simulink library "airlib"  (Simulink 3.00)
libraries: airlib x2
(part 1 of 2)
settings Model: LastModifiedBy=campa

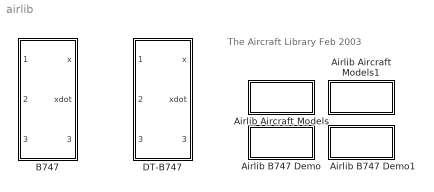
== system airlib ==
  note: The Aircraft Library
      | Feb 2003
  Airlib Aircraft Models : Subsystem
      settings: OpenFcn=airlibex
      mask Display: disp('Aircraft\nModels')
  Airlib Aircraft Models1 : Subsystem
      settings: OpenFcn=airgk
      mask Display: disp('General\nController')
  Airlib B747 Demo : Subsystem
      settings: OpenFcn=B747cl
      mask Display: disp('B747\nClosed Loop')
  Airlib B747 Demo1 : Subsystem
      settings: OpenFcn=fdcwind
      mask Display: disp('FDC\nwind model')
  B747 : Subsystem  mask(General Nonlinear Aircraft Model){GM1=[8.32   59.74   510.95   24675560  44876980   67383260   0   1315126  0   288772], CD_wind=[0.0164  0.2  0  0  0], CL_wind=[0.21  4.4  6.6  0.32  0.7], Cm_body=[0  -1   -20.5    -1.3    -2.7], CY_body=[0   -0.9    0     0     -0    0.12], Cl_body=[0    -0.16    -0.34   0.13    -0.013    0.008], Cn_body=[0    0.16   -0.026    -0.28     -0.0018   -0.1], x0=[150.148  0.0464959 0   0 0 0   0 0.0464959 0   0 0 61]}
      mask prompts: GM1 "Geometry and Mass : [cbar   b    S    Ix   Iy   Iz   Jxy  Jxz  Jyz  m]"; CD_wind "Aerodynamic D-Force Derivatives : [CD0 CDa CDq CDde CDih]"; CL_wind "Aerodynamic L-Force Derivatives : [CL0 CLa CLq CLde CLih]"; Cm_body "Aerodynamic Y-Moment Derivatives : [Cm0 Cma Cmq Cmde Cmih]"; CY_body "Aerodynamic Y-Force Derivatives : [CY0 CYb CYp CYr CYda CYdr]"; Cl_body "Aerodynamic X-moment Derivatives : [Cl0 Clb Clp Clr Clda Cldr]"; Cn_body "Aerodynamic Z-moment Derivatives : [Cn0 Cnb Cnp Cnr Cnda Cndr]"; x0 "Initial Condition x0 [v alpha beta p q r psi theta phi xe ye H]"
      mask help:
      | The first input contains the wind velocity and acceleration.
      |   The second input contains external forces and moments in body axis.
      |   The third input contains the deflections of elevators, ailerons, rudder,
      |   and flaps. For a list of outputs look under the mask.
      |   NB : The International measurement system (MKS) is adopted.
      mask init:
      | AM=zeros(6,19);
      | AM(1,[1 2 9 11 12])=reshape(CD_wind,1,5);
      | AM(3,[1 2 9 11 12])=reshape(CL_wind,1,5);
      | AM(5,[1 2 9 11 12])=reshape(Cm_body,1,5);
      | AM(2,[1 5 8 10 13 14])=reshape(CY_body,1,6);
      | AM(4,[1 5 8 10 13 14])=reshape(Cl_body,1,6);
      | AM(6,[1 5 8 10 13 14])=reshape(Cn_body,1,6);
      | 
      | Ix=GM1(4);Iy=GM1(5);Iz=GM1(6);
      | Jxy=GM1(7);Jxz=GM1(8);Jyz=GM1(9);
      | 
      | detI = Ix*Iy*Iz - 2*Jxy*Jxz*Jyz - Ix*Jyz^2 - Iy*Jxz^2 - Iz*Jxy^2;
      | I1   = Iy*Iz - Jyz^2;I2   = Jxy*Iz + Jyz*Jxz;
      | I3   = Jxy*Jyz + Iy*Jxz;I4   = Ix*Iz - Jxz^2;
      | I5   = Ix*Jyz + Jxy*Jxz;I6   = Ix*Iy - Jxy^2;
      | 
      | Pl  = I1/detI; Pm = I2/detI; Pn = I3/detI;
      | Ppp = -(Jxz*I2 - Jxy*I3)/detI;Ppq = (Jxz*I1 - Jyz*I2 - (Iy-Ix)*I3)/detI;
      | Ppr = -(Jxy*I1 + (Ix-Iz)*I2 - Jyz*I3)/detI;Pqq = (Jyz*I1 - Jxy*I3)/detI;
      | Pqr = -((Iz-Iy)*I1 - Jxy*I2 + Jxz*I3)/detI;Prr = -(Jyz*I1 - Jxz*I2)/detI;
      | 
      | Ql  = I2/detI; Qm = I4/detI; Qn = I5/detI;
      | Qpp = -(Jxz*I4 - Jxy*I5)/detI;Qpq = (Jxz*I2 - Jyz*I4 - (Iy-Ix)*I5)/detI;
      | Qpr = -(Jxy*I2 + (Ix-Iz)*I4 - Jyz*I5)/detI;Qqq = (Jyz*I2 - Jxy*I5)/detI;
      | Qqr = -((Iz-Iy)*I2 - Jxy*I4 + Jxz*I5)/detI;Qrr = -(Jyz*I2 - Jxz*I4)/detI;
      | 
      | Rl  = I3/detI; Rm = I5/detI; Rn = I6/detI;
      | Rpp = -(Jxz*I5 - Jxy*I6)/detI;
      | Rpq = (Jxz*I3 - Jyz*I5 - (Iy-Ix)*I6)/detI;
      | Rpr = -(Jxy*I3 + (Ix-Iz)*I5 - Jyz*I6)/detI;
      | Rqq = (Jyz*I3 - Jxy*I6)/detI;
      | Rqr = -((Iz-Iy)*I3 - Jxy*I5 + Jxz*I6)/detI;
      | Rrr = -(Jyz*I3 - Jxz*I5)/detI;
      | 
      | GM2 = [  Pl   Pm   Pn   Ppp  Ppq  Ppr  Pqq  Pqr  Prr ;
      |                Ql  Qm   Qn   Qpp  Qpq  Qpr  Qqq  Qqr  Qrr ;
      |                Rl  Rm   Rn   Rpp  Rpq  Rpr  Rqq  Rqr  Rrr ];
      | 
      | xfix=1;
      mask Help:
      | <p>
      | This block is a general nonlinear 6DOF aircraft model, with a very accurate built-in atmosphere model and constant aerodynamic derivatives.
      | The architecture of the block is largely based on the Aircraft block provided by the <A
      | HREF="http://www.mathworks.com/matlabcentral/fileexchange/loadFile.do?objectId=252&objectType=file">FDC toolbox</A> (Marc Rauw, 1993-2000).
      | </p>
      | <p>
      | The geometric and inertal data of the aircraft are entered as parameters in the first row of the mask. The other six rows contains the
      | non-dimensional aerodynamic derivatives. The last row is the initial state.
      | </p>
      | <p>
      | The first input contains the wind velocity and acceleration.
      | The second input contains external forces and moments in the aircraft body axis.
      | The third input contains the deflections of elevators, ailerons, rudder,
      | and flaps or stabilators. For a list of outputs look under the mask.
      | </p>
      | <p>
      | The control surface sign conventions are the same adopted in books such as Stevens-Lewis and Etkin, and in many flight simulators,
      | including the FDC toolbox. <br>
      | Specifically, positive elevator deflection causes negative pitching moment (Cmde &#60 0), positive rudder deflection causes negative yawing
      | moment (Cndr &#60 0), and positive aileron deflection causes negative rolling moment (Clda &#60 0). Another way to say the same thing is
      | that, the positive elevators deflection is Trailing Edge Down (TED), the positive rudder(s) deflection is Trailing Edge Left (TEL), and,
      | taking as TED the positive ailerons deflection, da=K*(da_right-da_left), with K usually equal to 1 (FDC) or 1/2.
      | </p>
      | <p>
      | Since this block is largely based on the FDC toolbox, i redirect you to the FDC Toolbox manual, for a good explanation of the underlying
      | components. Besides the mask and the fact that the aerodynamic derivatives are expressed in the stability axis, the only relevant difference
      | with the FDC toolbox is that in the computation of the aerodynamic forces, q is normalized as q*cbar/2V instead of q*cbar/V. The majority
      | of aeronautics books that i've seen use q*cbar/2V.
      | </p>
      | <p>
      | Please note that the International Measurement System is adopted. So, lengths are in meters, masses in Kg, and inertia moments in Kg*m^2.
      | Moreover, forces are in N, moments in N*m, accelerations in g, and angles in radians. For those that use the english system, here are some useful
      | conversion factors: <br>
      | 1 ft   = 0.3048 m, 1 lb   = 0.4536 Kg, 1 slug = 14.593903 Kg ,  1 slug*ft^2 = 1.355818 Kg*m^2
      | <br>
      | </p>
      | <p>
      | Finally, there is an <A HREF="http://www.aae.uiuc.edu/m-selig/apasim/Aircraft-uiuc.html">excellent source</A> of aircraft aerodynamic data
      | which is mantained by Michael S. Selig, Rob Deters, and Glen Dimock at the university of Urbana-Champaign. To use any of the given models
      | you just need to type the supplied aircraft data in the block mask.
      | </p>
      | <p>
      | <p>
      | December 2002, Giampiero Campa
      | </p>
      | </p>
      mask Display: disp('General\nAircraft\nModel')
  DT-B747 : Subsystem  mask(Discrete Time General Nonlinear Aircraft Model){GM1=[8.32   59.74   510.95   24675560  44876980   67383260   0   1315126  0   288772  0.05], CD_wind=[0.0164  0.2  0  0  0], CL_wind=[0.21  4.4  6.6  0.32  0.7], Cm_body=[0  -1   -20.5    -1.3    -2.7], CY_body=[0   -0.9    0     0     -0    0.12], Cl_body=[0    -0.16    -0.34   0.13    -0.013    0.008], Cn_body=[0    0.16   -0.026    -0.28     -0.0018   -0.1], x0=[150.148  0.0464959 0   0 0 0   0 0.0464959 0   0 0 61]}
      mask prompts: GM1 "Geometry, Mass, T : [cbar   b    S    Ix   Iy   Iz   Jxy  Jxz  Jyz  m  T]"; CD_wind "Aerodynamic D-Force Derivatives : [CD0 CDa CDq CDde CDih]"; CL_wind "Aerodynamic L-Force Derivatives : [CL0 CLa CLq CLde CLih]"; Cm_body "Aerodynamic Y-Moment Derivatives : [Cm0 Cma Cmq Cmde Cmih]"; CY_body "Aerodynamic Y-Force Derivatives : [CY0 CYb CYp CYr CYda CYdr]"; Cl_body "Aerodynamic X-moment Derivatives : [Cl0 Clb Clp Clr Clda Cldr]"; Cn_body "Aerodynamic Z-moment Derivatives : [Cn0 Cnb Cnp Cnr Cnda Cndr]"; x0 "Initial Condition x0 [v alpha beta p q r psi theta phi xe ye H]"
      mask help:
      | The first input contains the wind velocity and acceleration.
      |   The second input contains external forces and moments in body axis.
      |   The third input contains the deflections of elevators, ailerons, rudder,
      |   and flaps. For a list of outputs look under the mask.
      |   NB : The International measurement system (MKS) is adopted.
      mask init:
      | AM=zeros(6,19);
      | AM(1,[1 2 9 11 12])=reshape(CD_wind,1,5);
      | AM(3,[1 2 9 11 12])=reshape(CL_wind,1,5);
      | AM(5,[1 2 9 11 12])=reshape(Cm_body,1,5);
      | AM(2,[1 5 8 10 13 14])=reshape(CY_body,1,6);
      | AM(4,[1 5 8 10 13 14])=reshape(Cl_body,1,6);
      | AM(6,[1 5 8 10 13 14])=reshape(Cn_body,1,6);
      | 
      | Ix=GM1(4);Iy=GM1(5);Iz=GM1(6);
      | Jxy=GM1(7);Jxz=GM1(8);Jyz=GM1(9);
      | 
      | detI = Ix*Iy*Iz - 2*Jxy*Jxz*Jyz - Ix*Jyz^2 - Iy*Jxz^2 - Iz*Jxy^2;
      | I1   = Iy*Iz - Jyz^2;I2   = Jxy*Iz + Jyz*Jxz;
      | I3   = Jxy*Jyz + Iy*Jxz;I4   = Ix*Iz - Jxz^2;
      | I5   = Ix*Jyz + Jxy*Jxz;I6   = Ix*Iy - Jxy^2;
      | 
      | Pl  = I1/detI; Pm = I2/detI; Pn = I3/detI;
      | Ppp = -(Jxz*I2 - Jxy*I3)/detI;Ppq = (Jxz*I1 - Jyz*I2 - (Iy-Ix)*I3)/detI;
      | Ppr = -(Jxy*I1 + (Ix-Iz)*I2 - Jyz*I3)/detI;Pqq = (Jyz*I1 - Jxy*I3)/detI;
      | Pqr = -((Iz-Iy)*I1 - Jxy*I2 + Jxz*I3)/detI;Prr = -(Jyz*I1 - Jxz*I2)/detI;
      | 
      | Ql  = I2/detI; Qm = I4/detI; Qn = I5/detI;
      | Qpp = -(Jxz*I4 - Jxy*I5)/detI;Qpq = (Jxz*I2 - Jyz*I4 - (Iy-Ix)*I5)/detI;
      | Qpr = -(Jxy*I2 + (Ix-Iz)*I4 - Jyz*I5)/detI;Qqq = (Jyz*I2 - Jxy*I5)/detI;
      | Qqr = -((Iz-Iy)*I2 - Jxy*I4 + Jxz*I5)/detI;Qrr = -(Jyz*I2 - Jxz*I4)/detI;
      | 
      | Rl  = I3/detI; Rm = I5/detI; Rn = I6/detI;
      | Rpp = -(Jxz*I5 - Jxy*I6)/detI;
      | Rpq = (Jxz*I3 - Jyz*I5 - (Iy-Ix)*I6)/detI;
      | Rpr = -(Jxy*I3 + (Ix-Iz)*I5 - Jyz*I6)/detI;
      | Rqq = (Jyz*I3 - Jxy*I6)/detI;
      | Rqr = -((Iz-Iy)*I3 - Jxy*I5 + Jxz*I6)/detI;
      | Rrr = -(Jyz*I3 - Jxz*I5)/detI;
      | 
      | GM2 = [  Pl   Pm   Pn   Ppp  Ppq  Ppr  Pqq  Pqr  Prr ;
      |                Ql  Qm   Qn   Qpp  Qpq  Qpr  Qqq  Qqr  Qrr ;
      |                Rl  Rm   Rn   Rpp  Rpq  Rpr  Rqq  Rqr  Rrr ];
      | 
      | xfix=1;
      | T=GM1(11);
      mask Help:
      | <p>
      | This block is a general nonlinear 6DOF aircraft model, with a very accurate built-in atmosphere model and constant aerodynamic derivatives.
      | The architecture of the block is largely based on the Aircraft block provided by the <A
      | HREF="http://www.mathworks.com/matlabcentral/fileexchange/loadFile.do?objectId=252&objectType=file">FDC toolbox</A> (Marc Rauw, 1993-2000).
      | </p>
      | <p>
      | The geometric and inertal data of the aircraft are entered as parameters in the first row of the mask, sampling time is the last parameter. The other six rows contains the non-dimensional aerodynamic derivatives. The last row is the initial state.
      | </p>
      | <p>
      | The first input contains the wind velocity and acceleration.
      | The second input contains external forces and moments in the aircraft body axis.
      | The third input contains the deflections of elevators, ailerons, rudder,
      | and flaps or stabilators. For a list of outputs look under the mask.
      | </p>
      | <p>
      | The control surface sign conventions are the same adopted in books such as Stevens-Lewis and Etkin, and in many flight simulators,
      | including the FDC toolbox. <br>
      | Specifically, positive elevator deflection causes negative pitching moment (Cmde &#60 0), positive rudder deflection causes negative yawing
      | moment (Cndr &#60 0), and positive aileron deflection causes negative rolling moment (Clda &#60 0). Another way to say the same thing is
      | that, the positive elevators deflection is Trailing Edge Down (TED), the positive rudder(s) deflection is Trailing Edge Left (TEL), and,
      | taking as TED the positive ailerons deflection, da=K*(da_right-da_left), with K usually equal to 1 (FDC) or 1/2.
      | </p>
      | <p>
      | Since this block is largely based on the FDC toolbox, i redirect you to the FDC Toolbox manual, for a good explanation of the underlying
      | components. Besides the mask and the fact that the aerodynamic derivatives are expressed in the stability axis, the only relevant difference
      | with the FDC toolbox is that in the computation of the aerodynamic forces, q is normalized as q*cbar/2V instead of q*cbar/V. The majority
      | of aeronautics books that i've seen use q*cbar/2V.
      | </p>
      | <p>
      | Please note that the International Measurement System is adopted. So, lengths are in meters, masses in Kg, and inertia moments in Kg*m^2.
      | Moreover, forces are in N, moments in N*m, accelerations in g, and angles in radians. For those that use the english system, here are some useful
      | conversion factors: <br>
      | 1 ft   = 0.3048 m, 1 lb   = 0.4536 Kg, 1 slug = 14.593903 Kg ,  1 slug*ft^2 = 1.355818 Kg*m^2
      | <br>
      | </p>
      | <p>
      | Finally, there is an <A HREF="http://www.aae.uiuc.edu/m-selig/apasim/Aircraft-uiuc.html">excellent source</A> of aircraft aerodynamic data
      | which is mantained by Michael S. Selig, Rob Deters, and Glen Dimock at the university of Urbana-Champaign. To use any of the given models
      | you just need to type the supplied aircraft data in the block mask.
      | </p>
      | <p>
      | <p>
      | December 2002, Giampiero Campa
      | </p>
      | </p>
      mask Display: disp('Discrete\nTime\nGeneral\nAircraft\nModel')

== system airlib/Airlib Aircraft Models ==

== system airlib/Airlib Aircraft Models1 ==

== system airlib/Airlib B747 Demo ==

== system airlib/Airlib B747 Demo1 ==

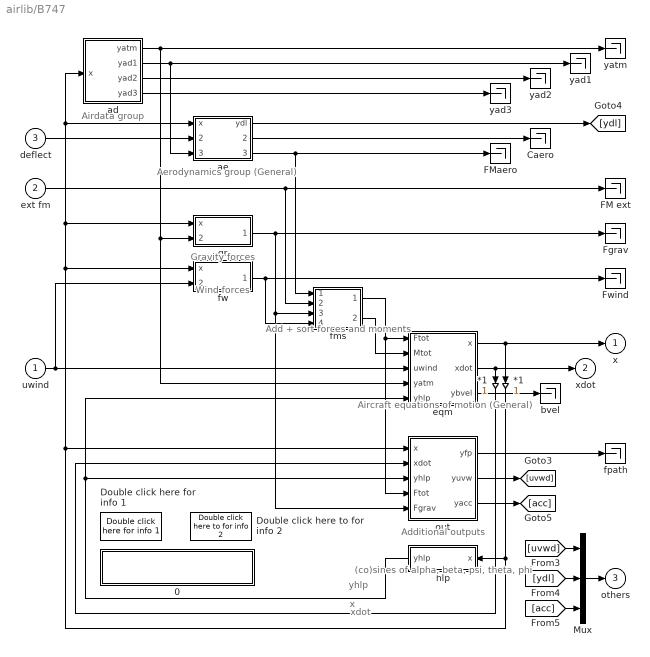
== system airlib/B747 ==
  note: Airdata group
  note: Add + sort
      | forces and
      | moments
  note: (co)sines of
      | alpha, beta,
      | psi, theta, phi
  note: Aerodynamics
      | group (General)
  note: Gravity forces
  note: Wind forces
  note: Aircraft equations
      | of motion (General)
  note: Additional outputs
  note: yhlp
  note: x
  note: xdot
  " uwind" : Inport  Port=1  PortWidth=-1  SampleTime=-1  DataType=auto
      settings: SignalType=auto
  ext fm : Inport  Port=2  PortWidth=-1  SampleTime=-1  DataType=auto
      settings: SignalType=auto
  deflect : Inport  Port=3  PortWidth=-1  SampleTime=-1  DataType=auto
      settings: SignalType=auto
  " *1" : Gain  Orientation=down  Gain=1  SaturateOnIntegerOverflow=on
  *1 : Gain  Orientation=down  Gain=1  SaturateOnIntegerOverflow=on
  0 : Subsystem
      mask Display: disp('AIRCRAFT, main level\nM.O. Rauw')
  Caero : Terminator
  Double click here for info 1 : airlib/DT-B747/Double click here for info 1
  Double click here to for info 2 : airlib/DT-B747/Double click here to for info 2
  FM ext : Terminator
  FMaero : Terminator
  Fgrav : Terminator
  Fwind : Terminator
  Mux : Mux  Inputs=[3 3 6]
  ad : Subsystem
  ae : Subsystem
  bvel : Terminator
  eqm : Subsystem
  fms : Subsystem
      mask Type: FMsort
      mask Description: Forces and Moments sorting block
      mask Display: disp('FMsort')
  fpath : Terminator
  fw : Subsystem  mask(fwind){m=GM1(10)}
      mask prompts: m "Mass of the aircraft [kg]:"
      mask help: Forces due to non-steady atmosphere.
      mask Display: disp('Fwind')
  gr : Subsystem  mask(Gravity){m=GM1(10)}
      mask prompts: m "Mass of the aircraft [kg]:"
      mask help: Gravity forces.
      mask Display: disp('Gravity')
  hlp : Subsystem  Orientation=left
      mask Type: Hlpfcn
      mask Description: Help sines and cosines
      mask Display: disp('hlpfcn')
  out : Subsystem
  yad1 : Terminator
  yad2 : Terminator
  yad3 : Terminator
  yatm : Terminator
  x : Outport  Port=1
  xdot : Outport  Port=2
  others : Outport  Port=3
  wires:
  Mux/1 -> others/1
  [acc] -> Mux/3
  [ydl] -> Mux/2
  [uvwd] -> Mux/1
  out/2(yuvw) -> [uvwd]
  fms/2(Mtot) -> eqm/2(Mtot)
  eqm/1(x) -> " *1"/1, x/1
  eqm/2(xdot) -> *1/1, xdot/1
  " *1"/1 -> ad/1(x), ae/1(x), gr/1(x), fw/1(x), out/1(x), hlp/1(x)
  gr/1(Fgrav) -> Fgrav/1, out/5(Fgrav), fms/3(Fgrav)
  *1/1 -> out/2(xdot)
  " uwind"/1 -> fw/2(uwind), eqm/3(uwind)
  hlp/1(yhlp) -> out/3(yhlp), eqm/5(yhlp)
  ae/3(FMaero) -> fms/1(FMaero), FMaero/1
  fw/1(Fwind) -> fms/4(Fwind), Fwind/1
  out/3(yacc) -> [acc]
  ad/1(yatm) -> yatm/1, gr/2(yatm), eqm/4(yatm)
  ad/3(yad2) -> yad2/1
  ad/2(yad1) -> yad1/1, ae/3(yad1)
  out/1(yfp) -> fpath/1
  eqm/3(ybvel) -> bvel/1
  ae/2(Caero) -> Caero/1
  ae/1(ydl) -> [ydl]
  ad/4(yad3) -> yad3/1
  deflect/1 -> ae/2(uaero)
  ext fm/1 -> FM ext/1, fms/2(FMprop)
  fms/1(Ftot) -> eqm/1(Ftot), out/4(Ftot)

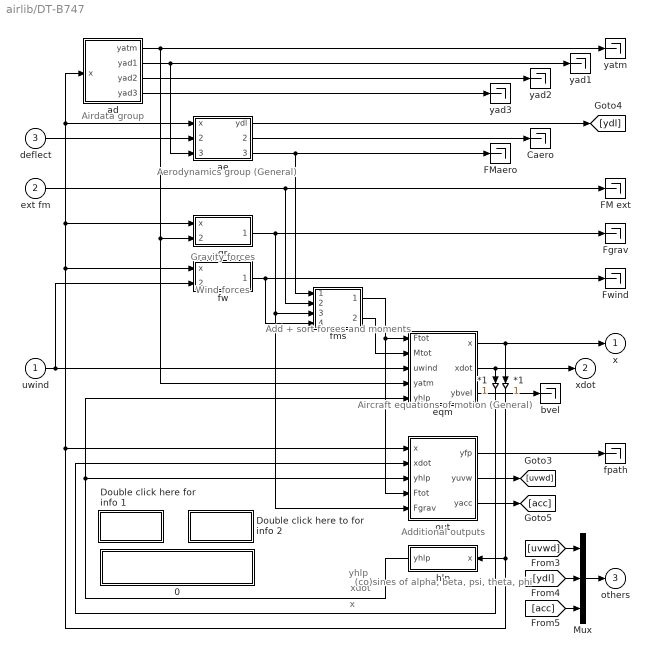
== system airlib/DT-B747 ==
  note: xdot
  note: x
  note: yhlp
  note: Additional outputs
  note: Aircraft equations
      | of motion (General)
  note: Wind forces
  note: Gravity forces
  note: Aerodynamics
      | group (General)
  note: (co)sines of
      | alpha, beta,
      | psi, theta, phi
  note: Add + sort
      | forces and
      | moments
  note: Airdata group
  " uwind" : Inport  Port=1  PortWidth=-1  SampleTime=-1  DataType=auto
      settings: SignalType=auto
  ext fm : Inport  Port=2  PortWidth=-1  SampleTime=-1  DataType=auto
      settings: SignalType=auto
  deflect : Inport  Port=3  PortWidth=-1  SampleTime=-1  DataType=auto
      settings: SignalType=auto
  " *1" : Gain  Orientation=down  Gain=1  SaturateOnIntegerOverflow=on
  *1 : Gain  Orientation=down  Gain=1  SaturateOnIntegerOverflow=on
  0 : Subsystem
      mask Display: disp('AIRCRAFT, main level\nM.O. Rauw')
  Caero : Terminator
  Double click here for info 1 : Subsystem
      mask Display: disp('Input\nSignals')
  Double click here to for info 2 : Subsystem
      mask Display: disp('Output\nSignals')
  FM ext : Terminator
  FMaero : Terminator
  Fgrav : Terminator
  Fwind : Terminator
  Mux : Mux  Inputs=[3 3 6]
  ad : Subsystem
  ae : Subsystem
  bvel : Terminator
  eqm : Subsystem
  fms : Subsystem
      mask Type: FMsort
      mask Description: Forces and Moments sorting block
      mask Display: disp('FMsort')
  fpath : Terminator
  fw : Subsystem  mask(fwind){m=GM1(10)}
      mask prompts: m "Mass of the aircraft [kg]:"
      mask help: Forces due to non-steady atmosphere.
      mask Display: disp('Fwind')
  gr : Subsystem  mask(Gravity){m=GM1(10)}
      mask prompts: m "Mass of the aircraft [kg]:"
      mask help: Gravity forces.
      mask Display: disp('Gravity')
  hlp : Subsystem  Orientation=left
      mask Type: Hlpfcn
      mask Description: Help sines and cosines
      mask Display: disp('hlpfcn')
  out : Subsystem
  yad1 : Terminator
  yad2 : Terminator
  yad3 : Terminator
  yatm : Terminator
  x : Outport  Port=1
  xdot : Outport  Port=2
  others : Outport  Port=3
  wires:
  fms/1(Ftot) -> out/4(Ftot), eqm/1(Ftot)
  ext fm/1 -> fms/2(FMprop), FM ext/1
  deflect/1 -> ae/2(uaero)
  ad/4(yad3) -> yad3/1
  ae/1(ydl) -> [ydl]
  ae/2(Caero) -> Caero/1
  eqm/3(ybvel) -> bvel/1
  out/1(yfp) -> fpath/1
  ad/2(yad1) -> ae/3(yad1), yad1/1
  ad/3(yad2) -> yad2/1
  ad/1(yatm) -> eqm/4(yatm), gr/2(yatm), yatm/1
  out/3(yacc) -> [acc]
  fw/1(Fwind) -> Fwind/1, fms/4(Fwind)
  ae/3(FMaero) -> FMaero/1, fms/1(FMaero)
  hlp/1(yhlp) -> eqm/5(yhlp), out/3(yhlp)
  " uwind"/1 -> eqm/3(uwind), fw/2(uwind)
  *1/1 -> out/2(xdot)
  gr/1(Fgrav) -> fms/3(Fgrav), out/5(Fgrav), Fgrav/1
  " *1"/1 -> hlp/1(x), out/1(x), fw/1(x), gr/1(x), ae/1(x), ad/1(x)
  eqm/2(xdot) -> xdot/1, *1/1
  eqm/1(x) -> x/1, " *1"/1
  fms/2(Mtot) -> eqm/2(Mtot)
  out/2(yuvw) -> [uvwd]
  [uvwd] -> Mux/1
  [ydl] -> Mux/2
  [acc] -> Mux/3
  Mux/1 -> others/1

== system airlib/B747/0 ==

== system airlib/B747/ad ==
  x : Inport  Port=1  PortWidth=-1  SampleTime=-1  DataType=auto
      settings: SignalType=auto
  0 : Subsystem
      mask Display: disp('AIRDATA GROUP (level 3)\nM.O. Rauw')
  ad1 : Subsystem
      mask Type: Airdata1
      mask Description: Basic airdata variables
      mask Display: disp('Airdata1')
  ad2 : Subsystem
      mask Type: Airdata2
      mask Description: More airdata variables
      mask Display: disp('Airdata2')
  ad3 : Subsystem  mask(Airdata3){cbar=GM1(1)}
      mask prompts: cbar "Mean aerodynamic chord [m]:"
      mask help: More airdata variables
      mask Display: disp('Airdata3')
  atm : Subsystem
      mask Type: Atmosph
      mask Description: Atmosphere variables
      mask Display: disp('Atmosph')
  yatm : Outport  Port=1
  yad1 : Outport  Port=2
  yad2 : Outport  Port=3
  yad3 : Outport  Port=4
  wires:
  ad1/1(yad1) -> ad3/3(yad1), ad2/2(yad1), yad1/1
  atm/1(yatm) -> ad3/2(yatm), ad2/1(yatm), ad1/2(yatm), yatm/1
  x/1 -> ad3/1(x), ad1/1(x), atm/1(x)
  ad3/1(yad3) -> yad3/1
  ad2/1(yad2) -> yad2/1

== system airlib/B747/ae ==
  x : Inport  Port=1  PortWidth=-1  SampleTime=-1  DataType=auto
      settings: SignalType=auto
  uaero : Inport  Port=2  PortWidth=-1  SampleTime=-1  DataType=auto
      settings: SignalType=auto
  yad1 : Inport  Port=3  PortWidth=-1  SampleTime=-1  DataType=auto
      settings: SignalType=auto
  0 : Subsystem
      mask Display: disp('AERODYNAMICS GROUP (level 3)\nM.O. Rauw')
  aero : Subsystem
      mask Type: Aeromod
      mask Description: Aerodynamic model of the DHC-2 'Beaver'.
      mask Display: disp('Aeromod\n(General)')
  dl : Subsystem  mask(Dimless){cbar=GM1(1), b=GM1(2)}
      mask prompts: cbar "Mean aerodynamic chord [m]:"; b "Wing span [m]:"
      mask help: Dimensionless rotational velocities.
      mask Display: disp('Dimless')
  fmdims : Subsystem  mask(FMdims){cbar=GM1(1), b=GM1(2), S=GM1(3)}
      mask prompts: cbar "Mean aerodynamic chord [m]:"; b "Wing span [m]:"; S "Wing surface [m^2]:"
      mask help:
      | Calculate forces and moments from
      | dimensionless derivatives.
      mask Display: disp('FMdims')
  ydl : Outport  Port=1
  Caero : Outport  Port=2
  FMaero : Outport  Port=3
  wires:
  fmdims/1(Forces and moments) -> FMaero/1
  yad1/1 -> fmdims/1(yad1)
  uaero/1 -> aero/2(uaero)
  x/1 -> aero/1(x), dl/1(x)
  dl/1(ydl) -> aero/3(ydl), ydl/1
  aero/1(Caero) -> fmdims/2(Force / moment derivatives), Caero/1

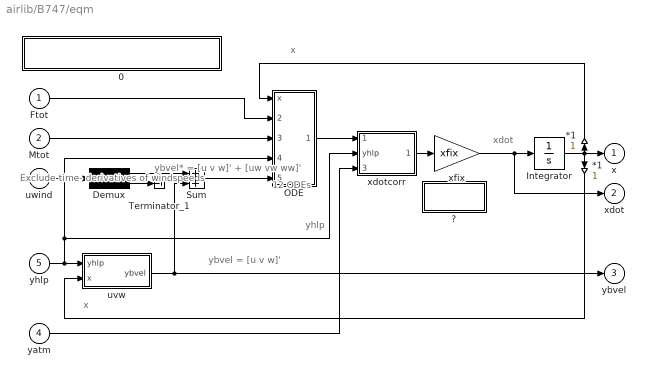
== system airlib/B747/eqm ==
  note: 12 ODEs
  note: ybvel = [u v w]'
  note: yhlp
  note: x
  note: x
  note: xdot
  note: ybvel* =
      | [u v w]' +
      | [uw vw ww]'
  note: Exclude time-
      | derivatives
      | of windspeeds
  Ftot : Inport  Port=1  PortWidth=-1  SampleTime=-1  DataType=auto
      settings: SignalType=auto
  Mtot : Inport  Port=2  PortWidth=-1  SampleTime=-1  DataType=auto
      settings: SignalType=auto
  uwind : Inport  Port=3  PortWidth=-1  SampleTime=-1  DataType=auto
      settings: SignalType=auto
  yatm : Inport  Port=4  PortWidth=-1  SampleTime=-1  DataType=auto
      settings: SignalType=auto
  yhlp : Inport  Port=5  PortWidth=-1  SampleTime=-1  DataType=auto
      settings: SignalType=auto
  " *1" : Gain  Orientation=up  Gain=1  SaturateOnIntegerOverflow=on
  *1 : Gain  Orientation=down  Gain=1  SaturateOnIntegerOverflow=on
  0 : Subsystem
      mask Display: disp('EQUATIONS OF MOTION (level 3)\nM.O. Rauw')
  "?" : Subsystem
      mask Display: disp('More info\nfor xfix')
  Demux : Demux  Outputs=[3 3]
  Integrator : Integrator  ExternalReset=none  InitialConditionSource=internal  InitialCondition=x0  LimitOutput=off  UpperSaturationLimit=inf  LowerSaturationLimit=-inf  ShowSaturationPort=off  ShowStatePort=off  AbsoluteTolerance=auto
  ODE : Subsystem
  Sum : Sum  Inputs=++  SaturateOnIntegerOverflow=on
  Terminator_1 : Terminator
  uvw : Subsystem
      mask Type: uvw
      mask Description:
      | Calculation of body-axes velocities
      | u, v, and w
      mask Display: disp('Body-axes\nvelocities')
  xdotcorr : Subsystem  mask(xdotcorr){b=GM1(2), S=GM1(3), m=GM1(10), CYbdot=AM(2,19)}
      mask prompts: b "Wing span [m]:"; S "Wing surface [m^2]:"; m "Mass of the aircraft [kg]:"; CYbdot "Stability-derivative CYbdot:"
      mask help:
      | Correction block to write state
      | equations for DHC-2 Beaver aircraft
      | explicitly.
      mask Display: disp('xdotcorr\n(General)')
  xfix : Gain  Gain=xfix  SaturateOnIntegerOverflow=on
  x : Outport  Port=1
  xdot : Outport  Port=2
  ybvel : Outport  Port=3
  wires:
  " *1"/1 -> ODE/1(x)
  xfix/1 -> xdot/1, Integrator/1
  Integrator/1 -> *1/1, " *1"/1, x/1
  *1/1 -> uvw/2(x)
  Mtot/1 -> ODE/3(Mtot)
  Ftot/1 -> ODE/2(Ftot)
  yatm/1 -> xdotcorr/3(yatm)
  xdotcorr/1(xdot corrected) -> xfix/1
  Demux/1 -> Sum/1
  uwind/1 -> Demux/1
  uvw/1(ybvel) -> Sum/2, ybvel/1
  Sum/1 -> ODE/5(ybvel*)
  ODE/1(xdot) -> xdotcorr/1(xdot uncorrected)
  yhlp/1 -> xdotcorr/2(yhlp), ODE/4(yhlp), uvw/1(yhlp)
  Demux/2 -> Terminator_1/1

== system airlib/B747/fms ==
  FMaero : Inport  Port=1  PortWidth=-1  SampleTime=-1  DataType=auto
      settings: SignalType=auto
  FMprop : Inport  Port=2  PortWidth=-1  SampleTime=-1  DataType=auto
      settings: SignalType=auto
  Fgrav : Inport  Port=3  PortWidth=-1  SampleTime=-1  DataType=auto
      settings: SignalType=auto
  Fwind : Inport  Port=4  PortWidth=-1  SampleTime=-1  DataType=auto
      settings: SignalType=auto
  0 : Subsystem
      mask Display: disp('FMSORT\nM.O. Rauw, October 1997')
  Demux : Demux  Outputs=[3 3]
  Demux1 : Demux  Outputs=[3 3]
  Sum1 : Sum  Inputs=++  SaturateOnIntegerOverflow=on
  Sum3 : Sum  Inputs=++++  SaturateOnIntegerOverflow=on
  Ftot : Outport  Port=1
  Mtot : Outport  Port=2
  wires:
  Fwind/1 -> Sum3/4
  Demux/1 -> Sum3/1
  Sum1/1 -> Mtot/1
  Sum3/1 -> Ftot/1
  Demux1/1 -> Sum3/2
  Fgrav/1 -> Sum3/3
  Demux/2 -> Sum1/1
  Demux1/2 -> Sum1/2
  FMprop/1 -> Demux1/1
  FMaero/1 -> Demux/1

== system airlib/B747/fw ==
  x : Inport  Port=1  PortWidth=-1  SampleTime=-1  DataType=auto
      settings: SignalType=auto
  uwind : Inport  Port=2  PortWidth=-1  SampleTime=-1  DataType=auto
      settings: SignalType=auto
  -Xw/m : Fcn  Expr=u[16] + u[5]*u[15] - u[6]*u[14]
  -Yw/m : Fcn  Expr=u[17] - u[4]*u[15] + u[6]*u[13]
  -Zw/m : Fcn  Expr=u[18] + u[4]*u[14] - u[5]*u[13]
  0 : Subsystem
      mask Display: disp('FWIND\nM.O. Rauw, Dec. 1996')
  Mux : Mux  Inputs=3
      settings: DisplayOption=none
  Mux1 : Mux  Inputs=[12 6]
      settings: DisplayOption=none
  gain : Gain  Gain=-m  SaturateOnIntegerOverflow=on
  Fwind : Outport  Port=1
  wires:
  -Zw/m/1 -> Mux/3
  -Xw/m/1 -> Mux/1
  -Yw/m/1 -> Mux/2
  Mux1/1 -> -Xw/m/1, -Zw/m/1, -Yw/m/1
  Mux/1 -> gain/1
  gain/1 -> Fwind/1
  x/1 -> Mux1/1
  uwind/1 -> Mux1/2

== system airlib/B747/gr ==
  x : Inport  Port=1  PortWidth=-1  SampleTime=-1  DataType=auto
      settings: SignalType=auto
  yatm : Inport  Port=2  PortWidth=-1  SampleTime=-1  DataType=auto
      settings: SignalType=auto
  0 : Subsystem
      mask Display: disp('GRAVITY\nM.O. Rauw, October 1997')
  Mux : Mux  Inputs=3
      settings: DisplayOption=none
  Mux1 : Mux  Inputs=[12 5]
      settings: DisplayOption=none
  Xgr : Fcn  Expr=-m*u[17]*sin(u[8])
  Ygr : Fcn  Expr=m*u[17]*cos(u[8])*sin(u[9])
  Zgr : Fcn  Expr=m*u[17]*cos(u[8])*cos(u[9])
  Fgrav : Outport  Port=1
  wires:
  yatm/1 -> Mux1/2
  x/1 -> Mux1/1
  Zgr/1 -> Mux/3
  Mux1/1 -> Zgr/1, Xgr/1, Ygr/1
  Mux/1 -> Fgrav/1
  Ygr/1 -> Mux/2
  Xgr/1 -> Mux/1

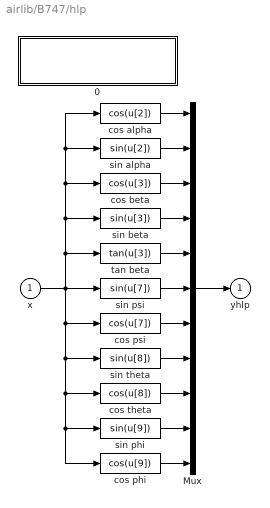
== system airlib/B747/hlp ==
  x : Inport  Port=1  PortWidth=-1  SampleTime=-1  DataType=auto
      settings: SignalType=auto
  0 : Subsystem
      mask Display: disp('HELP FUNCTIONS\n(often used sines and cosines)\nM.O. Rauw, October 1997')
  Mux : Mux  Inputs=11
      settings: DisplayOption=none
  cos alpha : Fcn  Expr=cos(u[2])
  cos beta : Fcn  Expr=cos(u[3])
  cos phi : Fcn  Expr=cos(u[9])
  cos psi : Fcn  Expr=cos(u[7])
  cos theta : Fcn  Expr=cos(u[8])
  sin alpha : Fcn  Expr=sin(u[2])
  sin beta : Fcn  Expr=sin(u[3])
  sin phi : Fcn  Expr=sin(u[9])
  sin psi : Fcn  Expr=sin(u[7])
  sin theta : Fcn  Expr=sin(u[8])
  tan beta : Fcn  Expr=tan(u[3])
  yhlp : Outport  Port=1
  wires:
  cos phi/1 -> Mux/11
  Mux/1 -> yhlp/1
  sin phi/1 -> Mux/10
  cos theta/1 -> Mux/9
  sin theta/1 -> Mux/8
  cos psi/1 -> Mux/7
  sin psi/1 -> Mux/6
  tan beta/1 -> Mux/5
  sin beta/1 -> Mux/4
  cos beta/1 -> Mux/3
  sin alpha/1 -> Mux/2
  cos alpha/1 -> Mux/1
  x/1 -> cos psi/1, cos phi/1, sin phi/1, cos theta/1, sin theta/1, tan beta/1, cos alpha/1, sin alpha/1, cos beta/1, sin beta/1, sin psi/1

== system airlib/B747/out ==
  note: Body-axes accelerations
      | and specific forces
  note: du/dt, dv/dt, dw/dt
      | (output equations!)
  note: Flightpath
      | variables
  x : Inport  Port=1  PortWidth=-1  SampleTime=-1  DataType=auto
      settings: SignalType=auto
  xdot : Inport  Port=2  PortWidth=-1  SampleTime=-1  DataType=auto
      settings: SignalType=auto
  yhlp : Inport  Port=3  PortWidth=-1  SampleTime=-1  DataType=auto
      settings: SignalType=auto
  Ftot : Inport  Port=4  PortWidth=-1  SampleTime=-1  DataType=auto
      settings: SignalType=auto
  Fgrav : Inport  Port=5  PortWidth=-1  SampleTime=-1  DataType=auto
      settings: SignalType=auto
  0 : Subsystem
      mask Display: disp('Additional outputs (level 3)\nM.O. Rauw')
  accel : Subsystem  mask(accel){m=GM1(10)}
      mask prompts: m "Mass of the aircraft [kg]:"
      mask help:
      | Body axes accelerations and
      | specific forces.
      mask Display: disp('Accel')
  fp : Subsystem  mask(Flpath){alpha0=x0(2)}
      mask prompts: alpha0 "Initial value of angle of attack, alpha0:"
      mask help: Flightpath related parameters.
      mask Display: disp('flpath')
  uvwdot : Subsystem
      mask Type: uvwdot
      mask Description: Calculation of du/dt, dv/dt, and dw/dt.
      mask Display: disp('uvwdot')
  yfp : Outport  Port=1
  yuvw : Outport  Port=2
  yacc : Outport  Port=3
  wires:
  Fgrav/1 -> accel/2(Fgrav)
  x/1 -> uvwdot/1(x), fp/1(x)
  xdot/1 -> uvwdot/2(xdot), fp/2(xdot)
  accel/1(yacc) -> yacc/1
  Ftot/1 -> accel/1(Ftot)
  yhlp/1 -> uvwdot/3(yhlp)
  uvwdot/1(yuvw =  [udot; vdot; wdot]) -> yuvw/1
  fp/1(yfp) -> yfp/1

== system airlib/DT-B747/0 ==

== system airlib/DT-B747/Double click here for info 1 ==
  note: 01 Uwind (m/s)
      | 02 Vwind (m/s)
      | 03 Wwind (m/s)
      | 04 Uwind_dot (m/s2)
      | 05 Vwind_dot (m/s2)
      | 06 Wwind_dot (m/s2)
      |
      | 07 Fx (N)
      | 08 Fy (N)
      | 09 Fz (N)
      | 10 Mx (N)
      | 11 My (N)
      | 12 Mz (N)
      |
      | 13 delta elevators (rad)
      | 14 delta ailerons (rad)
      | 15 delta rudder (rad)
      | 16 delta stabs/flaps (rad)

== system airlib/DT-B747/Double click here to for info 2 ==
  note: 01 v (m/s)
      | 02 alpha (rad)
      | 03 beta (rad)
      | 04 p (rad/s)
      | 05 q (rad/s)
      | 06 r  (rad/s)
      | 07 psi (rad)
      | 08 theta (rad)
      | 09 phi (rad)
      | 10 xe (m)
      | 11 ye (m)
      | 12 ze (m)
      |
      | 13 v dot (m/s2)
      | 14 alpha dot (rad/s)
      | 15 beta dot (rad/s)
      | 16 p dot (rad/s2)
      | 17 q dot (rad/s2)
      | 18 r dot (rad/s2)
      | 19 fi dot (rad/s)
      | 20 theta dot (rad/s)
      | 21 psi dot (rad/s)
      | 22 xe dot (m/s)
      | 23 ye dot (m/s)
      | 24 ze dot (m/s)
      |
      | 25 u dot (m/s2)
      | 26 v dot (m/s2)
      | 27 w dot (m/s2)
      | 28 pb/2v (rad)
      | 29 qc/v (rad)
      | 30 rb/v (rad)
      | 31 Ax (g)
      | 32 Ay (g)
      | 33 Az (g)
      | 34 ax (g)
      | 35 ay (g)
      | 36 az (g)

== system airlib/DT-B747/ad ==
  x : Inport  Port=1  PortWidth=-1  SampleTime=-1  DataType=auto
      settings: SignalType=auto
  0 : Subsystem
      mask Display: disp('AIRDATA GROUP (level 3)\nM.O. Rauw')
  ad1 : Subsystem
      mask Type: Airdata1
      mask Description: Basic airdata variables
      mask Display: disp('Airdata1')
  ad2 : Subsystem
      mask Type: Airdata2
      mask Description: More airdata variables
      mask Display: disp('Airdata2')
  ad3 : Subsystem  mask(Airdata3){cbar=GM1(1)}
      mask prompts: cbar "Mean aerodynamic chord [m]:"
      mask help: More airdata variables
      mask Display: disp('Airdata3')
  atm : Subsystem
      mask Type: Atmosph
      mask Description: Atmosphere variables
      mask Display: disp('Atmosph')
  yatm : Outport  Port=1
  yad1 : Outport  Port=2
  yad2 : Outport  Port=3
  yad3 : Outport  Port=4
  wires:
  ad2/1(yad2) -> yad2/1
  ad3/1(yad3) -> yad3/1
  x/1 -> atm/1(x), ad1/1(x), ad3/1(x)
  atm/1(yatm) -> yatm/1, ad1/2(yatm), ad2/1(yatm), ad3/2(yatm)
  ad1/1(yad1) -> yad1/1, ad2/2(yad1), ad3/3(yad1)

== system airlib/DT-B747/ae ==
  x : Inport  Port=1  PortWidth=-1  SampleTime=-1  DataType=auto
      settings: SignalType=auto
  uaero : Inport  Port=2  PortWidth=-1  SampleTime=-1  DataType=auto
      settings: SignalType=auto
  yad1 : Inport  Port=3  PortWidth=-1  SampleTime=-1  DataType=auto
      settings: SignalType=auto
  0 : Subsystem
      mask Display: disp('AERODYNAMICS GROUP (level 3)\nM.O. Rauw')
  aero : Subsystem
      mask Type: Aeromod
      mask Description: Aerodynamic model of the DHC-2 'Beaver'.
      mask Display: disp('Aeromod\n(General)')
  dl : Subsystem  mask(Dimless){cbar=GM1(1), b=GM1(2)}
      mask prompts: cbar "Mean aerodynamic chord [m]:"; b "Wing span [m]:"
      mask help: Dimensionless rotational velocities.
      mask Display: disp('Dimless')
  fmdims : Subsystem  mask(FMdims){cbar=GM1(1), b=GM1(2), S=GM1(3)}
      mask prompts: cbar "Mean aerodynamic chord [m]:"; b "Wing span [m]:"; S "Wing surface [m^2]:"
      mask help:
      | Calculate forces and moments from
      | dimensionless derivatives.
      mask Display: disp('FMdims')
  ydl : Outport  Port=1
  Caero : Outport  Port=2
  FMaero : Outport  Port=3
  wires:
  aero/1(Caero) -> Caero/1, fmdims/2(Force / moment derivatives)
  dl/1(ydl) -> ydl/1, aero/3(ydl)
  x/1 -> dl/1(x), aero/1(x)
  uaero/1 -> aero/2(uaero)
  yad1/1 -> fmdims/1(yad1)
  fmdims/1(Forces and moments) -> FMaero/1

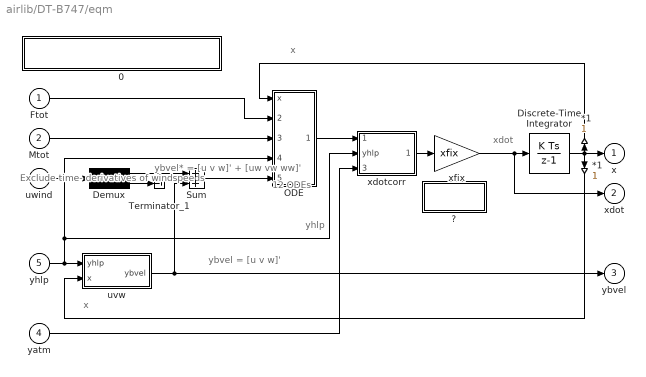
== system airlib/DT-B747/eqm ==
  note: Exclude time-
      | derivatives
      | of windspeeds
  note: ybvel* =
      | [u v w]' +
      | [uw vw ww]'
  note: xdot
  note: x
  note: x
  note: yhlp
  note: ybvel = [u v w]'
  note: 12 ODEs
  Ftot : Inport  Port=1  PortWidth=-1  SampleTime=-1  DataType=auto
      settings: SignalType=auto
  Mtot : Inport  Port=2  PortWidth=-1  SampleTime=-1  DataType=auto
      settings: SignalType=auto
  uwind : Inport  Port=3  PortWidth=-1  SampleTime=-1  DataType=auto
      settings: SignalType=auto
  yatm : Inport  Port=4  PortWidth=-1  SampleTime=-1  DataType=auto
      settings: SignalType=auto
  yhlp : Inport  Port=5  PortWidth=-1  SampleTime=-1  DataType=auto
      settings: SignalType=auto
  " *1" : Gain  Orientation=up  Gain=1  SaturateOnIntegerOverflow=on
  *1 : Gain  Orientation=down  Gain=1  SaturateOnIntegerOverflow=on
  0 : Subsystem
      mask Display: disp('EQUATIONS OF MOTION (level 3)\nM.O. Rauw')
  "?" : Subsystem
      mask Display: disp('More info\nfor xfix')
  Demux : Demux  Outputs=[3 3]
  Discrete-Time Integrator : DiscreteIntegrator  IntegratorMethod=ForwardEuler  ExternalReset=none  InitialConditionSource=internal  InitialCondition=x0  LimitOutput=off  UpperSaturationLimit=inf  LowerSaturationLimit=-inf  ShowSaturationPort=off  ShowStatePort=off  SampleTime=T
  ODE : Subsystem
  Sum : Sum  Inputs=++  SaturateOnIntegerOverflow=on
  Terminator_1 : Terminator
  uvw : Subsystem
      mask Type: uvw
      mask Description:
      | Calculation of body-axes velocities
      | u, v, and w
      mask Display: disp('Body-axes\nvelocities')
  xdotcorr : Subsystem  mask(xdotcorr){b=GM1(2), S=GM1(3), m=GM1(10), CYbdot=AM(2,19)}
      mask prompts: b "Wing span [m]:"; S "Wing surface [m^2]:"; m "Mass of the aircraft [kg]:"; CYbdot "Stability-derivative CYbdot:"
      mask help:
      | Correction block to write state
      | equations for DHC-2 Beaver aircraft
      | explicitly.
      mask Display: disp('xdotcorr\n(General)')
  xfix : Gain  Gain=xfix  SaturateOnIntegerOverflow=on
  x : Outport  Port=1
  xdot : Outport  Port=2
  ybvel : Outport  Port=3
  wires:
  Demux/2 -> Terminator_1/1
  yhlp/1 -> uvw/1(yhlp), ODE/4(yhlp), xdotcorr/2(yhlp)
  ODE/1(xdot) -> xdotcorr/1(xdot uncorrected)
  Sum/1 -> ODE/5(ybvel*)
  uvw/1(ybvel) -> ybvel/1, Sum/2
  uwind/1 -> Demux/1
  Demux/1 -> Sum/1
  xdotcorr/1(xdot corrected) -> xfix/1
  yatm/1 -> xdotcorr/3(yatm)
  Ftot/1 -> ODE/2(Ftot)
  Mtot/1 -> ODE/3(Mtot)
  *1/1 -> uvw/2(x)
  Discrete-Time Integrator/1 -> x/1, " *1"/1, *1/1
  xfix/1 -> Discrete-Time Integrator/1, xdot/1
  " *1"/1 -> ODE/1(x)

== system airlib/DT-B747/fms ==
  FMaero : Inport  Port=1  PortWidth=-1  SampleTime=-1  DataType=auto
      settings: SignalType=auto
  FMprop : Inport  Port=2  PortWidth=-1  SampleTime=-1  DataType=auto
      settings: SignalType=auto
  Fgrav : Inport  Port=3  PortWidth=-1  SampleTime=-1  DataType=auto
      settings: SignalType=auto
  Fwind : Inport  Port=4  PortWidth=-1  SampleTime=-1  DataType=auto
      settings: SignalType=auto
  0 : Subsystem
      mask Display: disp('FMSORT\nM.O. Rauw, October 1997')
  Demux : Demux  Outputs=[3 3]
  Demux1 : Demux  Outputs=[3 3]
  Sum1 : Sum  Inputs=++  SaturateOnIntegerOverflow=on
  Sum3 : Sum  Inputs=++++  SaturateOnIntegerOverflow=on
  Ftot : Outport  Port=1
  Mtot : Outport  Port=2
  wires:
  FMaero/1 -> Demux/1
  FMprop/1 -> Demux1/1
  Demux1/2 -> Sum1/2
  Demux/2 -> Sum1/1
  Fgrav/1 -> Sum3/3
  Demux1/1 -> Sum3/2
  Sum3/1 -> Ftot/1
  Sum1/1 -> Mtot/1
  Demux/1 -> Sum3/1
  Fwind/1 -> Sum3/4

== system airlib/DT-B747/fw ==
  x : Inport  Port=1  PortWidth=-1  SampleTime=-1  DataType=auto
      settings: SignalType=auto
  uwind : Inport  Port=2  PortWidth=-1  SampleTime=-1  DataType=auto
      settings: SignalType=auto
  -Xw/m : Fcn  Expr=u[16] + u[5]*u[15] - u[6]*u[14]
  -Yw/m : Fcn  Expr=u[17] - u[4]*u[15] + u[6]*u[13]
  -Zw/m : Fcn  Expr=u[18] + u[4]*u[14] - u[5]*u[13]
  0 : Subsystem
      mask Display: disp('FWIND\nM.O. Rauw, Dec. 1996')
  Mux : Mux  Inputs=3
      settings: DisplayOption=none
  Mux1 : Mux  Inputs=[12 6]
      settings: DisplayOption=none
  gain : Gain  Gain=-m  SaturateOnIntegerOverflow=on
  Fwind : Outport  Port=1
  wires:
  uwind/1 -> Mux1/2
  x/1 -> Mux1/1
  gain/1 -> Fwind/1
  Mux/1 -> gain/1
  Mux1/1 -> -Yw/m/1, -Zw/m/1, -Xw/m/1
  -Yw/m/1 -> Mux/2
  -Xw/m/1 -> Mux/1
  -Zw/m/1 -> Mux/3

== system airlib/DT-B747/gr ==
  x : Inport  Port=1  PortWidth=-1  SampleTime=-1  DataType=auto
      settings: SignalType=auto
  yatm : Inport  Port=2  PortWidth=-1  SampleTime=-1  DataType=auto
      settings: SignalType=auto
  0 : Subsystem
      mask Display: disp('GRAVITY\nM.O. Rauw, October 1997')
  Mux : Mux  Inputs=3
      settings: DisplayOption=none
  Mux1 : Mux  Inputs=[12 5]
      settings: DisplayOption=none
  Xgr : Fcn  Expr=-m*u[17]*sin(u[8])
  Ygr : Fcn  Expr=m*u[17]*cos(u[8])*sin(u[9])
  Zgr : Fcn  Expr=m*u[17]*cos(u[8])*cos(u[9])
  Fgrav : Outport  Port=1
  wires:
  Xgr/1 -> Mux/1
  Ygr/1 -> Mux/2
  Mux/1 -> Fgrav/1
  Mux1/1 -> Ygr/1, Xgr/1, Zgr/1
  Zgr/1 -> Mux/3
  x/1 -> Mux1/1
  yatm/1 -> Mux1/2

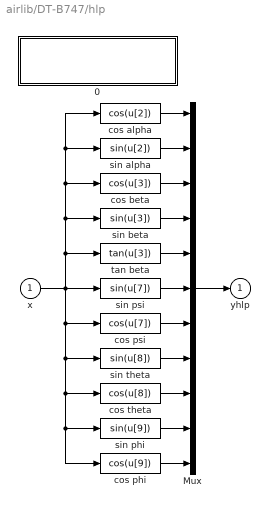
== system airlib/DT-B747/hlp ==
  x : Inport  Port=1  PortWidth=-1  SampleTime=-1  DataType=auto
      settings: SignalType=auto
  0 : Subsystem
      mask Display: disp('HELP FUNCTIONS\n(often used sines and cosines)\nM.O. Rauw, October 1997')
  Mux : Mux  Inputs=11
      settings: DisplayOption=none
  cos alpha : Fcn  Expr=cos(u[2])
  cos beta : Fcn  Expr=cos(u[3])
  cos phi : Fcn  Expr=cos(u[9])
  cos psi : Fcn  Expr=cos(u[7])
  cos theta : Fcn  Expr=cos(u[8])
  sin alpha : Fcn  Expr=sin(u[2])
  sin beta : Fcn  Expr=sin(u[3])
  sin phi : Fcn  Expr=sin(u[9])
  sin psi : Fcn  Expr=sin(u[7])
  sin theta : Fcn  Expr=sin(u[8])
  tan beta : Fcn  Expr=tan(u[3])
  yhlp : Outport  Port=1
  wires:
  x/1 -> sin psi/1, sin beta/1, cos beta/1, sin alpha/1, cos alpha/1, tan beta/1, sin theta/1, cos theta/1, sin phi/1, cos phi/1, cos psi/1
  cos alpha/1 -> Mux/1
  sin alpha/1 -> Mux/2
  cos beta/1 -> Mux/3
  sin beta/1 -> Mux/4
  tan beta/1 -> Mux/5
  sin psi/1 -> Mux/6
  cos psi/1 -> Mux/7
  sin theta/1 -> Mux/8
  cos theta/1 -> Mux/9
  sin phi/1 -> Mux/10
  Mux/1 -> yhlp/1
  cos phi/1 -> Mux/11

== system airlib/DT-B747/out ==
  note: Flightpath
      | variables
  note: du/dt, dv/dt, dw/dt
      | (output equations!)
  note: Body-axes accelerations
      | and specific forces
  x : Inport  Port=1  PortWidth=-1  SampleTime=-1  DataType=auto
      settings: SignalType=auto
  xdot : Inport  Port=2  PortWidth=-1  SampleTime=-1  DataType=auto
      settings: SignalType=auto
  yhlp : Inport  Port=3  PortWidth=-1  SampleTime=-1  DataType=auto
      settings: SignalType=auto
  Ftot : Inport  Port=4  PortWidth=-1  SampleTime=-1  DataType=auto
      settings: SignalType=auto
  Fgrav : Inport  Port=5  PortWidth=-1  SampleTime=-1  DataType=auto
      settings: SignalType=auto
  0 : Subsystem
      mask Display: disp('Additional outputs (level 3)\nM.O. Rauw')
  accel : Subsystem  mask(accel){m=GM1(10)}
      mask prompts: m "Mass of the aircraft [kg]:"
      mask help:
      | Body axes accelerations and
      | specific forces.
      mask Display: disp('Accel')
  fp : Subsystem  mask(Flpath){alpha0=x0(2)}
      mask prompts: alpha0 "Initial value of angle of attack, alpha0:"
      mask help: Flightpath related parameters.
      mask Display: disp('flpath')
  uvwdot : Subsystem
      mask Type: uvwdot
      mask Description: Calculation of du/dt, dv/dt, and dw/dt.
      mask Display: disp('uvwdot')
  yfp : Outport  Port=1
  yuvw : Outport  Port=2
  yacc : Outport  Port=3
  wires:
  fp/1(yfp) -> yfp/1
  uvwdot/1(yuvw =  [udot; vdot; wdot]) -> yuvw/1
  yhlp/1 -> uvwdot/3(yhlp)
  Ftot/1 -> accel/1(Ftot)
  accel/1(yacc) -> yacc/1
  xdot/1 -> fp/2(xdot), uvwdot/2(xdot)
  x/1 -> fp/1(x), uvwdot/1(x)
  Fgrav/1 -> accel/2(Fgrav)

== system airlib/B747/ad/0 ==

== system airlib/B747/ad/ad1 ==
  x : Inport  Port=1  PortWidth=-1  SampleTime=-1  DataType=auto
      settings: SignalType=auto
  yatm : Inport  Port=2  PortWidth=-1  SampleTime=-1  DataType=auto
      settings: SignalType=auto
  0 : Subsystem
      mask Display: disp('AIRDATA1\nM.O. Rauw, October 1997')
  M : Fcn  Expr=u[2]/u[1]
  Mux : Mux  Inputs=[1 12]
      settings: DisplayOption=none
  Mux1 : Mux  Inputs=[12 5]
      settings: DisplayOption=none
  Mux2 : Mux  Inputs=3
      settings: DisplayOption=none
  a : Fcn  Expr=sqrt(401.8743*u[3])
  qdyn : Fcn  Expr=0.5*u[13]*u[1]^2
  yad1 : Outport  Port=1
  wires:
  yatm/1 -> Mux1/2, a/1
  x/1 -> Mux1/1, Mux/2
  Mux/1 -> M/1
  Mux1/1 -> qdyn/1
  M/1 -> Mux2/2
  a/1 -> Mux2/1, Mux/1
  qdyn/1 -> Mux2/3
  Mux2/1 -> yad1/1

== system airlib/B747/ad/ad2 ==
  yatm : Inport  Port=1  PortWidth=-1  SampleTime=-1  DataType=auto
      settings: SignalType=auto
  yad1 : Inport  Port=2  PortWidth=-1  SampleTime=-1  DataType=auto
      settings: SignalType=auto
  0 : Subsystem
      mask Display: disp('AIRDATA2\nM.O. Rauw, October 1997')
  Mux : Mux  Inputs=[5 3]
      settings: DisplayOption=none
  Mux1 : Mux  Inputs=3
      settings: DisplayOption=none
  Vc : Fcn  Expr=sqrt(579000*((1+u[1]/101325)^(1/3.5)-1))
  Ve : Fcn  Expr=sqrt(u[8] * 1.63265)
  qc : Fcn  Expr=u[2] * ((1+0.2*u[7]^2)^3.5-1)
  yad2 : Outport  Port=1
  wires:
  Mux1/1 -> yad2/1
  qc/1 -> Mux1/1, Vc/1
  Vc/1 -> Mux1/3
  Ve/1 -> Mux1/2
  Mux/1 -> Ve/1, qc/1
  yatm/1 -> Mux/1
  yad1/1 -> Mux/2

== system airlib/B747/ad/ad3 ==
  x : Inport  Port=1  PortWidth=-1  SampleTime=-1  DataType=auto
      settings: SignalType=auto
  yatm : Inport  Port=2  PortWidth=-1  SampleTime=-1  DataType=auto
      settings: SignalType=auto
  yad1 : Inport  Port=3  PortWidth=-1  SampleTime=-1  DataType=auto
      settings: SignalType=auto
  0 : Subsystem
      mask Display: disp('AIRDATA3\nM.O. Rauw, October 1997')
  Mux : Mux  Inputs=3
      settings: DisplayOption=none
  Mux1 : Mux  Inputs=[12 5 3]
      settings: DisplayOption=none
  Re : Fcn  Expr=(u[13]*u[1])/u[16]
  Tt : Fcn  Expr=u[15] * (1+0.2*u[19]^2)
  cbar : Gain  Gain=cbar  SaturateOnIntegerOverflow=on
  yad3 : Outport  Port=1
  wires:
  cbar/1 -> Mux/3
  Tt/1 -> Mux/1
  Mux/1 -> yad3/1
  Mux1/1 -> Tt/1, Re/1
  Re/1 -> cbar/1, Mux/2
  x/1 -> Mux1/1
  yatm/1 -> Mux1/2
  yad1/1 -> Mux1/3

== system airlib/B747/ad/atm ==
  x : Inport  Port=1  PortWidth=-1  SampleTime=-1  DataType=auto
      settings: SignalType=auto
  0 : Subsystem
      mask Display: disp('ATMOSPH\nM.O. Rauw, October 1997')
  Mux : Mux  Inputs=2
      settings: DisplayOption=none
  Mux1 : Mux  Inputs=[2 1]
      settings: DisplayOption=none
  Mux2 : Mux  Inputs=5
      settings: DisplayOption=none
  T : Fcn  Expr=288.15 - 0.0065*u[12]
  g : Fcn  Expr=9.80665*(6371020/(6371020+u[12]))^2
  mu : Fcn  Expr=(1.458*10^(-6)*u[2]^1.5)/(u[2]+110.4)
  ps : Fcn  Expr=101325*(u[2]/288.15)^(u[1]/1.86584)
  rho : Fcn  Expr=u[3]/(287.053*u[2])
  yatm : Outport  Port=1
  wires:
  mu/1 -> Mux2/4
  Mux2/1 -> yatm/1
  Mux1/1 -> rho/1
  rho/1 -> Mux2/1
  g/1 -> Mux2/5, Mux/1
  T/1 -> Mux2/3, Mux/2
  ps/1 -> Mux2/2, Mux1/2
  Mux/1 -> ps/1, mu/1, Mux1/1
  x/1 -> g/1, T/1

== system airlib/B747/ae/0 ==

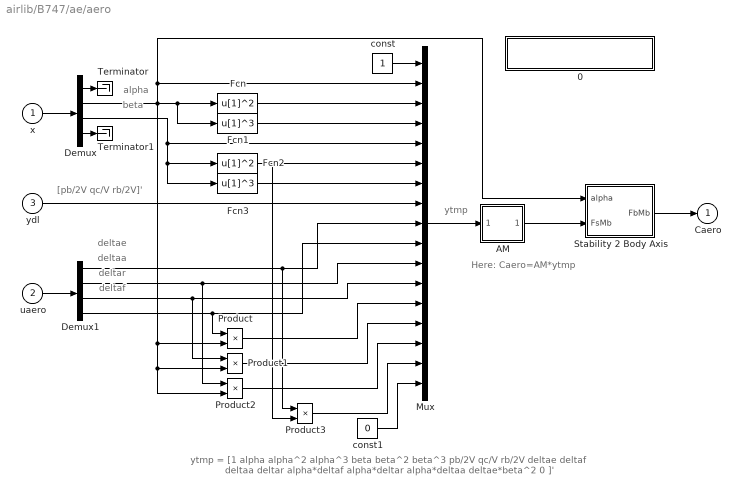
== system airlib/B747/ae/aero ==
  note: Here: Caero=AM*ytmp
  note: ytmp
  note: alpha
  note: deltaf
  note: deltar
  note: deltaa
  note: deltae
  note: beta
  note: [pb/2V qc/V rb/2V]'
  note: ytmp = [1  alpha  alpha^2  alpha^3  beta  beta^2  beta^3  pb/2V  qc/V  rb/2V  deltae
      | deltaf  deltaa  deltar  alpha*deltaf  alpha*deltar  alpha*deltaa  deltae*beta^2  0 ]'
  x : Inport  Port=1  PortWidth=-1  SampleTime=-1  DataType=auto
      settings: SignalType=auto
  uaero : Inport  Port=2  PortWidth=-1  SampleTime=-1  DataType=auto
      settings: SignalType=auto
  ydl : Inport  Port=3  PortWidth=-1  SampleTime=-1  DataType=auto
      settings: SignalType=auto
  0 : Subsystem
      mask Display: disp('AEROMOD\nM.O. Rauw, October 1997')
  "AM " : Subsystem  mask(State Space){M=AM}
      mask prompts: M "Matrix"
      mask Display: disp('Matrix\nGain')
  Demux : Demux  Outputs=[1 1 1 9]
  Demux1 : Demux  Outputs=4
  Fcn : Fcn  Expr=u[1]^2
  Fcn1 : Fcn  Expr=u[1]^3
  Fcn2 : Fcn  Expr=u[1]^2
  Fcn3 : Fcn  Expr=u[1]^3
  Mux : Mux  Inputs=[1 1 1 1 1 1 1 3 1 1 1 1 1 1 1 1 1]
      settings: DisplayOption=none
  Product{,1..3} (4 alike) : Product  Inputs=2  SaturateOnIntegerOverflow=on
  Stability 2 Body Axis : Subsystem
  Terminator : Terminator
  Terminator1 : Terminator
  const : Constant  Value=1
  const1 : Constant  Value=0
  Caero : Outport  Port=1
  wires:
  "AM "/1(Out1) -> Stability 2 Body Axis/2(FsMb)
  Stability 2 Body Axis/1(FbMb) -> Caero/1
  Mux/1 -> "AM "/1(In1)
  x/1 -> Demux/1
  Fcn/1 -> Mux/3
  Fcn1/1 -> Mux/4
  uaero/1 -> Demux1/1
  Fcn3/1 -> Mux/7
  Product/1 -> Mux/13
  Demux1/3 -> Product1/1, Mux/12
  Demux1/2 -> Product2/1, Mux/11
  Demux/3 -> Fcn3/1, Fcn2/1, Mux/5
  Demux/2 -> Stability 2 Body Axis/1(alpha), Mux/2, Product2/2, Product1/2, Product/2, Fcn1/1, Fcn/1
  Demux1/4 -> Product/1, Mux/10
  Fcn2/1 -> Product3/2, Mux/6
  Demux1/1 -> Product3/1, Mux/9
  Product1/1 -> Mux/14
  Product2/1 -> Mux/15
  Product3/1 -> Mux/16
  ydl/1 -> Mux/8
  const/1 -> Mux/1
  const1/1 -> Mux/17
  Demux/1 -> Terminator/1
  Demux/4 -> Terminator1/1

== system airlib/B747/ae/dl ==
  x : Inport  Port=1  PortWidth=-1  SampleTime=-1  DataType=auto
      settings: SignalType=auto
  0 : Subsystem
      mask Display: disp('DIMLESS\nM.O. Rauw, October 1997')
  Mux : Mux  Inputs=3
      settings: DisplayOption=none
  pb/2V : Fcn  Expr=0.5 * u[4] * b / u[1]
  qc/2V : Fcn  Expr=0.5* u[5] * cbar / u[1]
  rb/2V : Fcn  Expr=0.5 * u[6] * b / u[1]
  ydl : Outport  Port=1
  wires:
  x/1 -> pb/2V/1, rb/2V/1, qc/2V/1
  Mux/1 -> ydl/1
  rb/2V/1 -> Mux/3
  qc/2V/1 -> Mux/2
  pb/2V/1 -> Mux/1

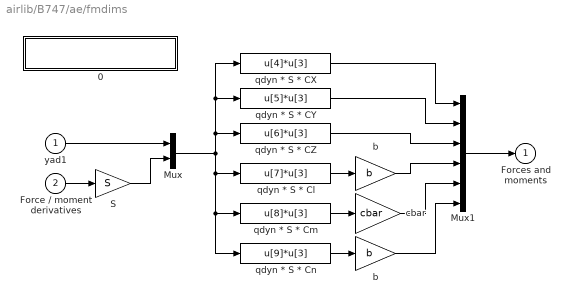
== system airlib/B747/ae/fmdims ==
  yad1 : Inport  Port=1  PortWidth=-1  SampleTime=-1  DataType=auto
      settings: SignalType=auto
  Force / moment derivatives : Inport  Port=2  PortWidth=-1  SampleTime=-1  DataType=auto
      settings: SignalType=auto
  0 : Subsystem
      mask Display: disp('FMDIMS\nM.O. Rauw, October 1997')
  Mux : Mux  Inputs=[3 6]
      settings: DisplayOption=none
  Mux1 : Mux  Inputs=6
      settings: DisplayOption=none
  S : Gain  Gain=S  SaturateOnIntegerOverflow=on
  b : Gain  Gain=b  SaturateOnIntegerOverflow=on
  "b " : Gain  Gain=b  SaturateOnIntegerOverflow=on
  cbar : Gain  Gain=cbar  SaturateOnIntegerOverflow=on
  qdyn * S * CX : Fcn  Expr=u[4]*u[3]
  qdyn * S * CY : Fcn  Expr=u[5]*u[3]
  qdyn * S * CZ : Fcn  Expr=u[6]*u[3]
  qdyn * S * Cl : Fcn  Expr=u[7]*u[3]
  qdyn * S * Cm : Fcn  Expr=u[8]*u[3]
  qdyn * S * Cn : Fcn  Expr=u[9]*u[3]
  Forces and moments : Outport  Port=1
  wires:
  b/1 -> Mux1/4
  qdyn * S * CZ/1 -> Mux1/3
  S/1 -> Mux/2
  qdyn * S * CY/1 -> Mux1/2
  qdyn * S * CX/1 -> Mux1/1
  yad1/1 -> Mux/1
  qdyn * S * Cn/1 -> "b "/1
  qdyn * S * Cm/1 -> cbar/1
  qdyn * S * Cl/1 -> b/1
  Mux/1 -> qdyn * S * Cn/1, qdyn * S * Cm/1, qdyn * S * Cl/1, qdyn * S * CY/1, qdyn * S * CX/1, qdyn * S * CZ/1
  Force / moment derivatives/1 -> S/1
  cbar/1 -> Mux1/5
  "b "/1 -> Mux1/6
  Mux1/1 -> Forces and moments/1

== system airlib/B747/eqm/0 ==

== system airlib/B747/eqm/? ==
